simulink model "pwm_motor"  (R2017a)
settings: Solver=FixedStepAuto  StartTime=0.0  StopTime=tf  FixedStep=1e-6  RelTol=1e-3
values from neighbouring files (symbols this model uses):
  A = double(subs(A_sym, symbs, vals))    [load_params.m]
  alpha_ = 0.5    [load_params.m]    (also in ss_value.m = alphas(i))
  B = double(subs(B_sym, symbs, vals))    [load_params.m]
  C = double(subs(C_sym, symbs, vals))    [load_params.m]    (also in load_pwm_avg_pred_controller.m = sysd.c; load_pwm_pred_controller.m = sysd.c)
  D = double(subs(D_sym, symbs, vals))    [load_params.m]
  max_val = 2    [load_params.m]
  min_val = 0    [load_params.m]
  T = 1e-3    (= 0.001)    [load_params.m]
  x0 = [0; 0]    [sim_controlled_system.m]
settings Model: Creator=brunolnetto  LastModifiedBy=brunolnetto

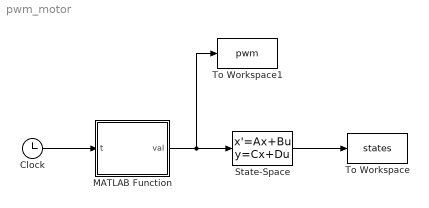
== system pwm_motor ==
  Clock : Clock
  MATLAB Function : MATLAB Function  TreatAsAtomicUnit=on
  State-Space : StateSpace  A=A  B=B  C=C  D=D  X0=x0
  To Workspace : ToWorkspace  VariableName=states  SaveFormat=Structure With Time  SampleTime=-1
  To Workspace1 : ToWorkspace  VariableName=pwm  SaveFormat=Structure With Time  SampleTime=-1
  wires:
  State-Space/1 -> To Workspace/1
  MATLAB Function/1(val) -> To Workspace1/1, State-Space/1
  Clock/1 -> MATLAB Function/1(t)

== matlab function pwm_motor/MATLAB Function ==
  data: t input; val output; max_val parameter; min_val parameter; alpha_ parameter; T parameter
function val = pwm_signal(t, max_val, min_val, alpha_, T)
    persistent t0;
    if(isempty(t0))
        t0 = 0;
    end
    
    if(t == 0)
        t0 = 0;
    end
    
    if(t - t0 > T)
        t0 = t;
    end
    
    t_i = t - t0;
    
    if(t_i < alpha_*T)
        val = max_val;
    else
        val = min_val;
    end
end
